simulink model "single_phase_WPT_v3"  (R2021a)
settings: Solver=FixedStepDiscrete  StartTime=0.0  StopTime=Tfinal  FixedStep=SampleTime  RelTol=1e-3
InitFcn:
  | param
values from neighbouring files (symbols this model uses):
  C_DCA = 1e-6    (= 1e-06)    [param.m]
  C_DCB = 1e-6    (= 1e-06)    [param.m]
  C_DCC = 1e-6    (= 1e-06)    [param.m]
  Cp = 28e-9    (= 2.8e-08)    [param.m]
  Cs = 120e-9    (= 1.2e-07)    [param.m]
  ESRA = 1e-7    (= 1e-07)    [param.m]
  ESRB = 1e-7    (= 1e-07)    [param.m]
  ESRC = 1e-7    (= 1e-07)    [param.m]
  f_motor = 50    [param.m]
  Lmotor = 30e-3    (= 0.03)    [param.m]
  Lp = 205e-6    (= 0.000205)    [param.m]
  Ls = 50e-6    (= 5e-05)    [param.m]
  LSource = 1e-9    (= 1e-09)    [param.m]
  M = 40e-6    (= 4e-05)    [param.m]
  ma = 0:0.01:1    [analitik_calculation.m]    (also in analytical_v2.m; param.m = 0.6)
  RL = 13    [param.m]
  Rmotor = 13    [param.m]
  RSource = 0.001    [param.m]
  SampleTime = 1e-8    (= 1e-08)    [param.m]
  Tfinal = 0.08    [param.m]
  VDC = 50    [param.m]
undefined symbols (not defined in the file or in its folder): ESLA, ESLB
libraries: spsSeriesRLCBranchLib x17, spsCurrentMeasurementLib x15, spsVoltageMeasurementLib x9, spsMosfetLib x6, spsTriangleGeneratorLib x3, spsDCVoltageSourceLib x1, eeStairGenerator x1, spsVariableResistorLib x1, spspowerguiLib x1
settings Model: Creator=enes_  LastModifiedBy=enes_
settings SolverCC: AlgebraicLoopSolver=TrustRegion
settings DataIOCC: ReturnWorkspaceOutputs=off
settings DebuggingCC: SFMachineParentedDataDiag=warning  ArithmeticOperatorsInVariantConditions=warning
settings SFSimCC: SimUseLocalCustomCode=off  CustomCodeUndefinedFunction=UseInterfaceOnly
settings RTWCC: RTWUseLocalCustomCode=off

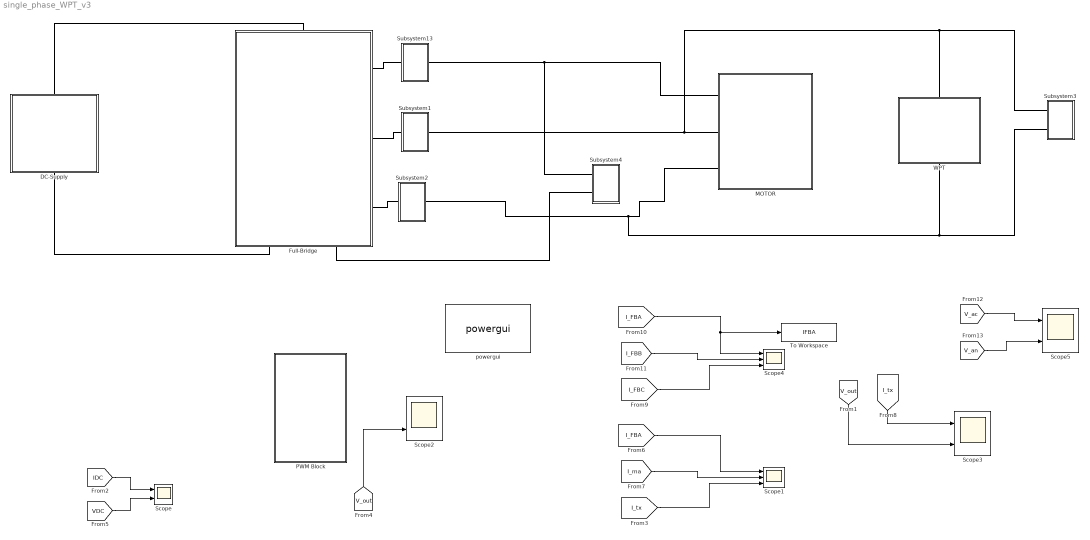
== system single_phase_WPT_v3 ==
  DC-Supply : Subsystem
  Full-Bridge : Subsystem
      settings: PortSchema="{\"entries\":[{\"content\":{\"sides\":[{\"content\":{\"connectorIds\":[]},\"type\":\"ConnectorPlacement.EquallySpacedRectSide\",\"uuid\":\"92c2640b-bb56-47f8-9c41-2323b38839f8\"},{\"content\":{\"connectorIds\":[\"RConn1\",\"RConn2\",\"RConn3\"],\"side\":\"RIGHT\"},\"type\":\"ConnectorPlacement.EquallySpacedRectSide\",\"uuid\":\"0b5c90a1-e2e1-4478-84c9-834496a6568e\"},{\"content\":{\"connectorIds\":[\"LConn1\"],\"side\":\"TOP\"},\"type\":\"ConnectorPlacement.EquallySpacedRectSide\",\"uuid\":\"1c803fb0-9096-4a7d-b495-aabd35d72306\"},{\"content\":{\"connectorIds\":[\"RConn4\",\"RConn5\"],\"side\":\"BOTTOM\"},\"type\":\"ConnectorPlacement.EquallySpacedRectSide\",\"uuid\":\"5a2d766c-8c3f-4943-ab0f-0e1988e2f8d8\"},{\"content\":{\"connectorIds\":[],\"side\":\"HIDDEN\"},\"type\":\"ConnectorPlacement.EquallySpacedRectSide\",\"uuid\":\"8868c32c-a67f-4887-a91d-dc24242eaee2\"}]},\"type\":\"ConnectorPlacement.EquallySpacedConnector\",\"uuid\":\"a3546067-6216-40b0-bae0-9d71271c5112\"}],\"packageUris\":[\"http://schema.mathworks.com/mf0/Connector/R2020b\"],\"version\":\"1.0\"}"
  MOTOR : Subsystem
      settings: PortSchema="{\"entries\":[{\"content\":{\"sides\":[{\"content\":{\"connectorIds\":[]},\"type\":\"ConnectorPlacement.EquallySpacedRectSide\",\"uuid\":\"27af0988-5d70-46f2-9f63-66e4679735d7\"},{\"content\":{\"connectorIds\":[],\"side\":\"RIGHT\"},\"type\":\"ConnectorPlacement.EquallySpacedRectSide\",\"uuid\":\"9d673fb6-38db-4110-ad66-771dcf318fba\"},{\"content\":{\"connectorIds\":[\"LConn1\",\"LConn2\",\"LConn3\"],\"side\":\"TOP\"},\"type\":\"ConnectorPlacement.EquallySpacedRectSide\",\"uuid\":\"44eb7bd4-c702-4f50-84c2-cb9d75020b5b\"},{\"content\":{\"connectorIds\":[],\"side\":\"HIDDEN\"},\"type\":\"ConnectorPlacement.EquallySpacedRectSide\",\"uuid\":\"ba714e9b-5efc-4dbb-add8-803f06cf9de0\"}]},\"type\":\"ConnectorPlacement.EquallySpacedConnector\",\"uuid\":\"a2219d53-abb4-437b-a840-c37860cec52f\"}],\"packageUris\":[\"http://schema.mathworks.com/mf0/Connector/R2020b\"],\"version\":\"1.0\"}"
  PWM Block : Subsystem
  Scope{,2..3,5} (4 alike) : Scope  NumInputPorts=2
  Scope1 : Scope  NumInputPorts=3
  Scope4 : Scope  NumInputPorts=3
  Subsystem1 : Subsystem
  Subsystem13 : Subsystem
  Subsystem2 : Subsystem
  Subsystem3 : Subsystem
  Subsystem4 : Subsystem
  To Workspace : ToWorkspace  VariableName=IFBA  SaveFormat=Timeseries  SampleTime=-1
  WPT : Subsystem
  powergui : spspowerguiLib/powergui  Priority=1  SimulationMode=Discrete  SampleTime=SampleTime  frequency=60  Iterations=50  frequencyindice=0  Pbase=100e6  ErrMax=1e-4  UnitsV=kV  UnitsW=MW  buscounter=0  FunctionMessages=off  echomessages=off  EnableUseOfTLC=off  CurrentSourceSwitches=off  DisableSnubberDevices=off  DisableRonSwitches=off  DisableVfSwitches=off  DisplayEquations=off  AutomaticDiscreteSolvers=off  SolverType=Tustin/Backward Euler (TBE)  Interpol=off  ExternalGateDelay=off  methode=off  Ts=100  x0status=blocks  SPID=on  SwTol=0  HookPort=off  NonlinearTolerance=1e-4  nMaxIteration=100  ContinueOnMaxIteration=off  RestoreLinks=warning  ResistiveCurrentMeasurement=off  Frange=[1e3:1e3:240e3]  Ylog=off  Xlog=on  ShowGrid=off  save=off  variable=ZData  structure=ScopeData2  ZoomFFT=off  StartTime=0.0005  cycles=800  DisplayStyle=1  fundamental=80000  FreqAxis=on  MaxFrequency=100e3  frequencyindicesteady=1  RmsSteady=1  display=off
  wires:
  [IDC] -> Scope/1
  [VDC] -> Scope/2
  [I_FBA] -> Scope1/1
  [I_ma] -> Scope1/2
  [I_tx] -> Scope1/3
  [V_out] -> Scope2/2
  ? -> Scope2/1
  [V_out] -> Scope3/2
  [I_tx] -> Scope3/1
  [I_FBB] -> Scope4/2
  [I_FBA] -> To Workspace/1, Scope4/1
  [I_FBC] -> Scope4/3
  [V_ac] -> Scope5/1
  [V_an] -> Scope5/2
  connections:
  DC-Supply/LConn1 -- Full-Bridge/LConn1
  DC-Supply/RConn1 -- Full-Bridge/RConn4
  Subsystem13/RConn1 -- Full-Bridge/RConn1
  MOTOR/LConn1 -- Subsystem13/LConn1 -- Subsystem4/LConn1
  Full-Bridge/RConn3 -- Subsystem2/RConn1
  Subsystem1/RConn1 -- Full-Bridge/RConn2
  WPT/LConn1 -- Subsystem3/LConn1 -- MOTOR/LConn2 -- Subsystem1/LConn1
  MOTOR/LConn3 -- WPT/RConn1 -- Subsystem3/LConn2 -- Subsystem2/LConn1
  Subsystem4/LConn2 -- Full-Bridge/RConn5

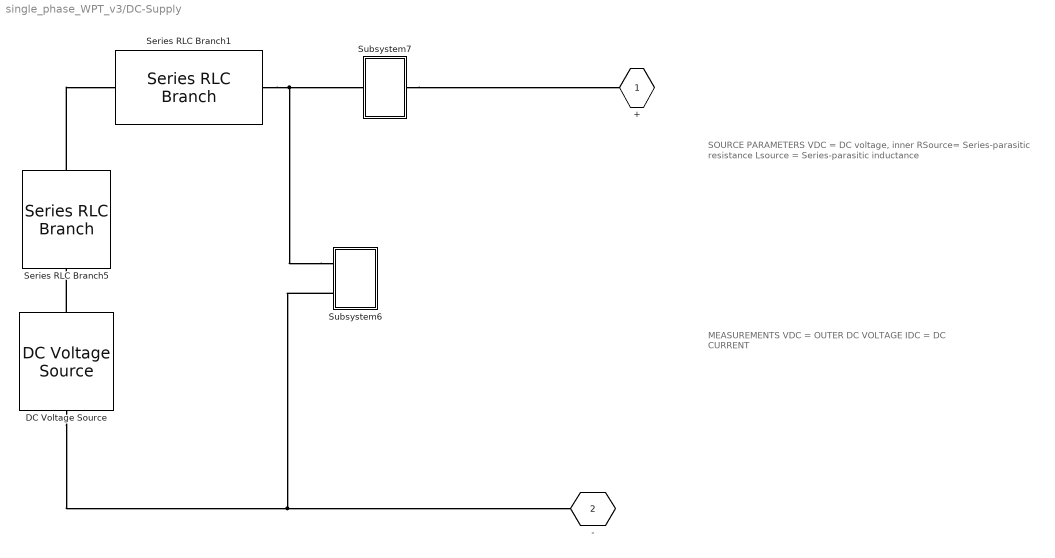
== system single_phase_WPT_v3/DC-Supply ==
  note: SOURCE PARAMETERS
      | VDC = DC voltage, inner
      | RSource= Series-parasitic resistance
      | Lsource = Series-parasitic inductance
  note: MEASUREMENTS
      | VDC = OUTER DC VOLTAGE
      | IDC = DC CURRENT
  DC Voltage Source : spsDCVoltageSourceLib/DC Voltage Source  Amplitude=VDC  Measurements=None
  Series RLC Branch1 : spsSeriesRLCBranchLib/Series RLC Branch  LConnTagsString=__new0  RConnTagsString=__new0  BranchType=L  Resistance=LSource  Inductance=LSource  SetiL0=off  InitialCurrent=0  Capacitance=0.01  Setx0=off  InitialVoltage=0  Measurements=None
  Series RLC Branch5 : spsSeriesRLCBranchLib/Series RLC Branch  LConnTagsString=__new0  RConnTagsString=__new0  BranchType=R  Resistance=RSource  Inductance=ESLA  SetiL0=off  InitialCurrent=0  Capacitance=0.01  Setx0=off  InitialVoltage=0  Measurements=None
  Subsystem6 : Subsystem
  Subsystem7 : Subsystem
  + : PMIOPort  Side=Left
  - : PMIOPort  Port=2  Side=Right
  connections:
  Series RLC Branch5/LConn1 -- Series RLC Branch1/RConn1
  DC Voltage Source/LConn1 -- Subsystem6/LConn2 -- -/RConn1
  Subsystem6/LConn1 -- Subsystem7/RConn1 -- Series RLC Branch1/LConn1
  DC Voltage Source/RConn1 -- Series RLC Branch5/RConn1
  Subsystem7/LConn1 -- +/RConn1

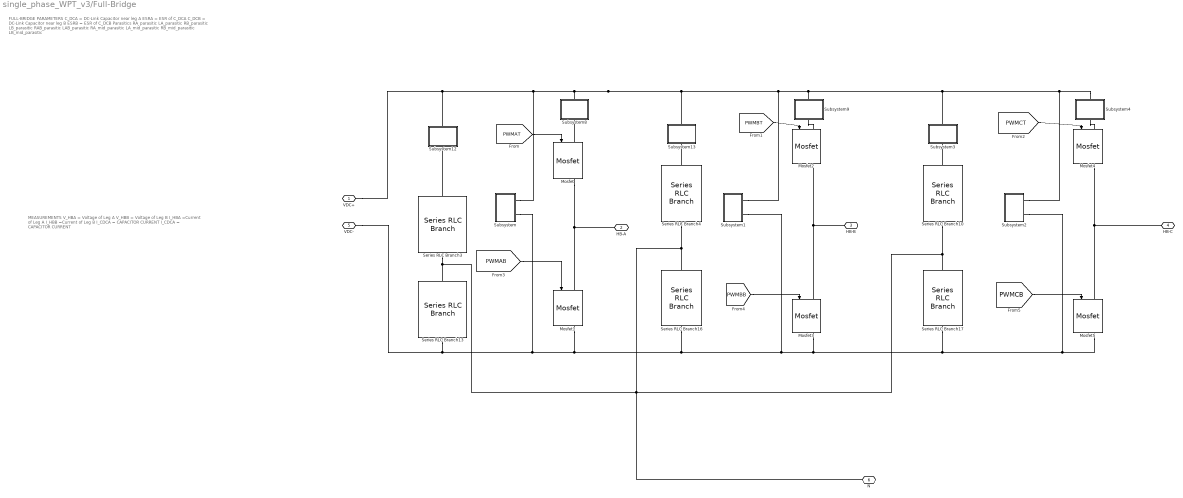
== system single_phase_WPT_v3/Full-Bridge ==
  note: MEASUREMENTS
      | V_HBA = Voltage of Leg A
      | V_HBB = Voltage of Leg B
      | I_HBA =Current of Leg A
      | I_HBB =Current of Leg B
      | I_CDCA = CAPACITOR CURRENT
      | I_CDCA = CAPACITOR CURRENT
  note: FULL-BRIDGE PARAMETERS
      | C_DCA = DC-Link Capacitor near leg A
      | ESRA = ESR of C_DCA
      | C_DCB = DC-Link Capacitor near leg B
      | ESRB = ESR of C_DCB
      | Parasitics
      | RA_parasitic
      | LA_parasitic
      | RB_parasitic
      | LB_parasitic
      | RAB_parasitic
      | LAB_parasitic
      | RA_mid_parasitic
      | LA_mid_parasitic
      | RB_mid_parasitic
      | LB_mid_parasitic
  Mosfet{,1..5} (6 alike) : spsMosfetLib/Mosfet  Ron=0.1  Lon=0  Rd=0.01  Vfd=0  IC=0  Rs=1e5  Cs=inf  Measurements=on
  Series RLC Branch10 : spsSeriesRLCBranchLib/Series RLC Branch  LConnTagsString=__new0  RConnTagsString=__new0  BranchType=C  Resistance=ESRC  Inductance=ESLB  SetiL0=off  InitialCurrent=0  Capacitance=C_DCC  Setx0=off  InitialVoltage=0  Measurements=None
  Series RLC Branch13 : spsSeriesRLCBranchLib/Series RLC Branch  LConnTagsString=__new0  RConnTagsString=__new0  BranchType=C  Resistance=ESRA  Inductance=ESLA  SetiL0=off  InitialCurrent=0  Capacitance=C_DCA  Setx0=off  InitialVoltage=0  Measurements=None
  Series RLC Branch16 : spsSeriesRLCBranchLib/Series RLC Branch  LConnTagsString=__new0  RConnTagsString=__new0  BranchType=C  Resistance=ESRB  Inductance=ESLB  SetiL0=off  InitialCurrent=0  Capacitance=C_DCB  Setx0=off  InitialVoltage=0  Measurements=None
  Series RLC Branch17 : spsSeriesRLCBranchLib/Series RLC Branch  LConnTagsString=__new0  RConnTagsString=__new0  BranchType=C  Resistance=ESRC  Inductance=ESLB  SetiL0=off  InitialCurrent=0  Capacitance=C_DCC  Setx0=off  InitialVoltage=0  Measurements=None
  Series RLC Branch3 : spsSeriesRLCBranchLib/Series RLC Branch  LConnTagsString=__new0  RConnTagsString=__new0  BranchType=C  Resistance=ESRA  Inductance=ESLA  SetiL0=off  InitialCurrent=0  Capacitance=C_DCA  Setx0=off  InitialVoltage=0  Measurements=None
  Series RLC Branch4 : spsSeriesRLCBranchLib/Series RLC Branch  LConnTagsString=__new0  RConnTagsString=__new0  BranchType=C  Resistance=ESRB  Inductance=ESLB  SetiL0=off  InitialCurrent=0  Capacitance=C_DCB  Setx0=off  InitialVoltage=0  Measurements=None
  Subsystem : Subsystem
  Subsystem1 : Subsystem
  Subsystem12 : Subsystem
  Subsystem13 : Subsystem
  Subsystem2 : Subsystem
  Subsystem3 : Subsystem
  Subsystem4 : Subsystem
  Subsystem8 : Subsystem
  Subsystem9 : Subsystem
  VDC+ : PMIOPort  Side=Left
  HB-A : PMIOPort  Port=2  Side=Right
  HB-B : PMIOPort  Port=3  Side=Right
  HB-C : PMIOPort  Port=4  Side=Right
  VDC- : PMIOPort  Port=5  Side=Right
  N : PMIOPort  Port=6  Side=Right
  wires:
  [PWMAB] -> Mosfet1/1
  [PWMAT] -> Mosfet/1
  [PWMBB] -> Mosfet3/1
  [PWMBT] -> Mosfet2/1
  [PWMCT] -> Mosfet4/1
  [PWMCB] -> Mosfet5/1
  connections:
  Subsystem4/RConn1 -- VDC+/RConn1 -- Subsystem12/RConn1 -- Subsystem/LConn1 -- Subsystem8/RConn1 -- Subsystem13/RConn1 -- Subsystem1/LConn1 -- Subsystem9/RConn1 -- Subsystem3/RConn1 -- Subsystem2/LConn1
  Subsystem9/LConn1 -- Mosfet2/LConn1
  Series RLC Branch4/LConn1 -- Subsystem13/LConn1
  Series RLC Branch3/LConn1 -- Subsystem12/LConn1
  HB-B/RConn1 -- Mosfet2/RConn1 -- Mosfet3/LConn1
  Mosfet/LConn1 -- Subsystem8/LConn1
  Subsystem2/LConn2 -- Mosfet5/RConn1 -- Series RLC Branch17/RConn1 -- Series RLC Branch16/RConn1 -- Series RLC Branch13/RConn1 -- VDC-/RConn1 -- Subsystem/LConn2 -- Mosfet1/RConn1 -- Subsystem1/LConn2 -- Mosfet3/RConn1
  HB-A/RConn1 -- Mosfet/RConn1 -- Mosfet1/LConn1
  Series RLC Branch10/LConn1 -- Subsystem3/LConn1
  HB-C/RConn1 -- Mosfet4/RConn1 -- Mosfet5/LConn1
  Subsystem4/LConn1 -- Mosfet4/LConn1
  Series RLC Branch10/RConn1 -- Series RLC Branch16/LConn1 -- Series RLC Branch4/RConn1 -- Series RLC Branch13/LConn1 -- Series RLC Branch3/RConn1 -- N/RConn1 -- Series RLC Branch17/LConn1

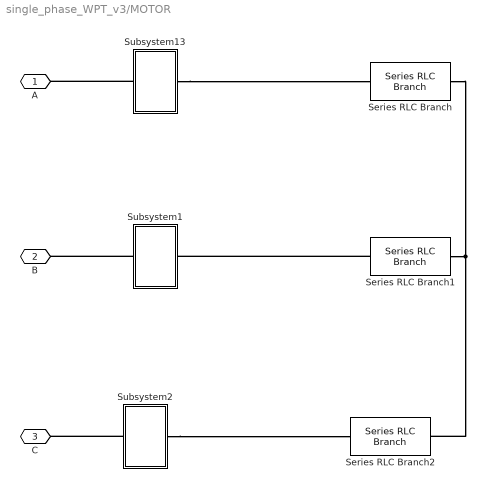
== system single_phase_WPT_v3/MOTOR ==
  Series RLC Branch : spsSeriesRLCBranchLib/Series RLC Branch  LConnTagsString=__new0  RConnTagsString=__new0  BranchType=RL  Resistance=Rmotor  Inductance=Lmotor  SetiL0=off  InitialCurrent=0  Capacitance=1e-6  Setx0=off  InitialVoltage=0  Measurements=None
  Series RLC Branch1 : spsSeriesRLCBranchLib/Series RLC Branch  LConnTagsString=__new0  RConnTagsString=__new0  BranchType=RL  Resistance=Rmotor  Inductance=Lmotor  SetiL0=off  InitialCurrent=0  Capacitance=1e-6  Setx0=off  InitialVoltage=0  Measurements=None
  Series RLC Branch2 : spsSeriesRLCBranchLib/Series RLC Branch  LConnTagsString=__new0  RConnTagsString=__new0  BranchType=RL  Resistance=Rmotor  Inductance=Lmotor  SetiL0=off  InitialCurrent=0  Capacitance=1e-6  Setx0=off  InitialVoltage=0  Measurements=None
  Subsystem1 : Subsystem
  Subsystem13 : Subsystem
  Subsystem2 : Subsystem
  A : PMIOPort  Side=Left
  B : PMIOPort  Port=2  Side=Left
  C : PMIOPort  Port=3  Side=Left
  connections:
  Subsystem13/LConn1 -- Series RLC Branch/LConn1
  Subsystem13/RConn1 -- A/RConn1
  Subsystem1/RConn1 -- B/RConn1
  Subsystem2/RConn1 -- C/RConn1
  Series RLC Branch1/LConn1 -- Subsystem1/LConn1
  Subsystem2/LConn1 -- Series RLC Branch2/LConn1
  Series RLC Branch/RConn1 -- Series RLC Branch2/RConn1 -- Series RLC Branch1/RConn1

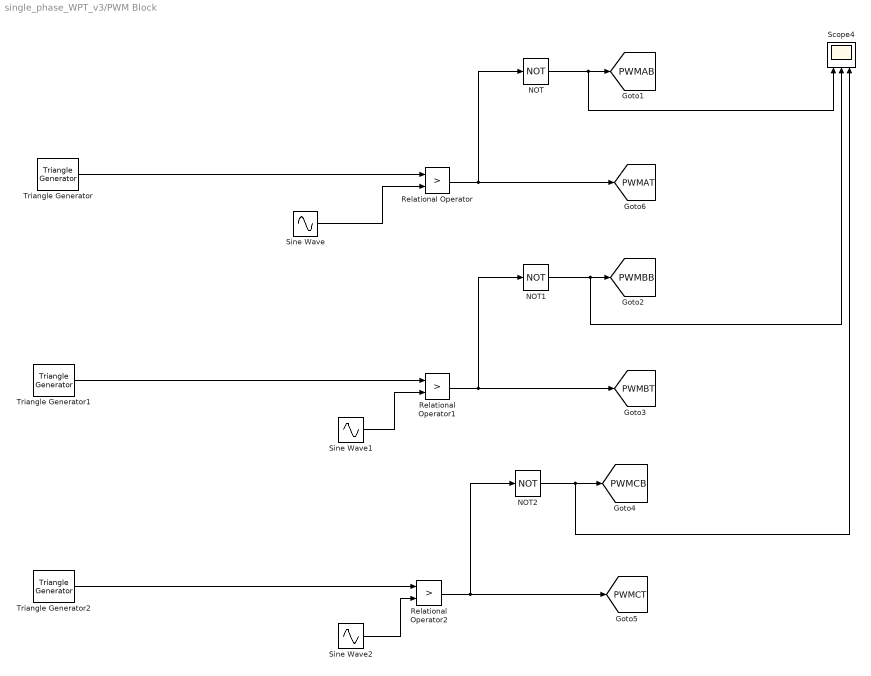
== system single_phase_WPT_v3/PWM Block ==
  NOT : Logic  Operator=NOT  IconShape=distinctive  AllPortsSameDT=off  OutDataTypeStr=boolean
  NOT1 : Logic  Operator=NOT  IconShape=distinctive  AllPortsSameDT=off  OutDataTypeStr=boolean
  NOT2 : Logic  Operator=NOT  IconShape=distinctive  AllPortsSameDT=off  OutDataTypeStr=boolean
  Relational Operator : RelationalOperator  Operator=>  OutDataTypeStr=boolean  RndMeth=Simplest
  Relational Operator1 : RelationalOperator  Operator=>  OutDataTypeStr=boolean  RndMeth=Simplest
  Relational Operator2 : RelationalOperator  Operator=>  OutDataTypeStr=boolean  RndMeth=Simplest
  Scope4 : Scope  NumInputPorts=3
  Sine Wave : Sin  Amplitude=ma  Frequency=f_motor*2*pi  SampleTime=0
  Sine Wave1 : Sin  Amplitude=ma  Frequency=f_motor*2*pi  Phase=-2*pi/3  SampleTime=0
  Sine Wave2 : Sin  Amplitude=ma  Frequency=f_motor*2*pi  Phase=2*pi/3  SampleTime=0
  Triangle Generator : spsTriangleGeneratorLib/Triangle Generator  Freq=80e3  Phase=0  Ts=SampleTime
  Triangle Generator1 : spsTriangleGeneratorLib/Triangle Generator  Freq=80e3  Phase=-120  Ts=SampleTime
  Triangle Generator2 : spsTriangleGeneratorLib/Triangle Generator  Freq=80e3  Phase=120  Ts=SampleTime
  tag scope: PWMAB=global, PWMAT=global, PWMBB=global, PWMBT=global, PWMCB=global, PWMCT=global
  wires:
  NOT/1 -> Scope4/1, [PWMAB]
  Relational Operator/1 -> NOT/1, [PWMAT]
  Relational Operator1/1 -> NOT1/1, [PWMBT]
  NOT2/1 -> [PWMCB], Scope4/3
  Relational Operator2/1 -> NOT2/1, [PWMCT]
  Sine Wave/1 -> Relational Operator/2
  Sine Wave2/1 -> Relational Operator2/2
  Sine Wave1/1 -> Relational Operator1/2
  NOT1/1 -> Scope4/2, [PWMBB]
  Triangle Generator/1 -> Relational Operator/1
  Triangle Generator1/1 -> Relational Operator1/1
  Triangle Generator2/1 -> Relational Operator2/1

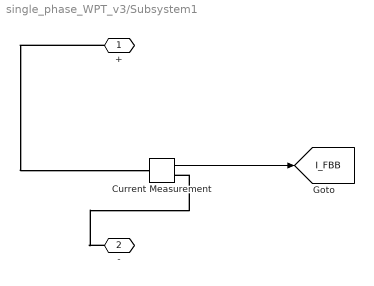
== system single_phase_WPT_v3/Subsystem1 ==
  Current Measurement : spsCurrentMeasurementLib/Current Measurement  PhasorSimulation=off  OutputType=Complex  PSBequivalent=0
  + : PMIOPort  Side=Right
  - : PMIOPort  Port=2  Side=Left
  tag scope: I_FBB=global
  wires:
  Current Measurement/1 -> [I_FBB]
  connections:
  +/RConn1 -- Current Measurement/LConn1
  -/RConn1 -- Current Measurement/RConn1

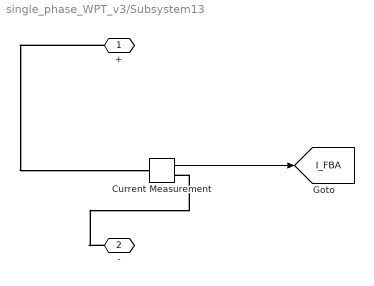
== system single_phase_WPT_v3/Subsystem13 ==
  Current Measurement : spsCurrentMeasurementLib/Current Measurement  PhasorSimulation=off  OutputType=Complex  PSBequivalent=0
  + : PMIOPort  Side=Right
  - : PMIOPort  Port=2  Side=Left
  tag scope: I_FBA=global
  wires:
  Current Measurement/1 -> [I_FBA]
  connections:
  +/RConn1 -- Current Measurement/LConn1
  -/RConn1 -- Current Measurement/RConn1

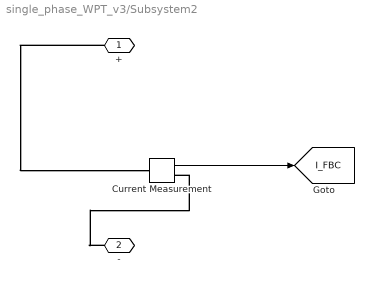
== system single_phase_WPT_v3/Subsystem2 ==
  Current Measurement : spsCurrentMeasurementLib/Current Measurement  PhasorSimulation=off  OutputType=Complex  PSBequivalent=0
  + : PMIOPort  Side=Right
  - : PMIOPort  Port=2  Side=Left
  tag scope: I_FBC=global
  wires:
  Current Measurement/1 -> [I_FBC]
  connections:
  +/RConn1 -- Current Measurement/LConn1
  -/RConn1 -- Current Measurement/RConn1

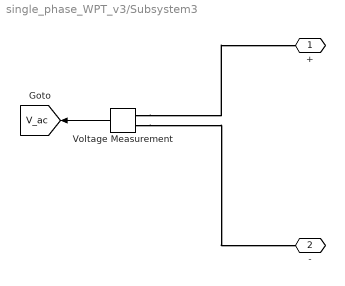
== system single_phase_WPT_v3/Subsystem3 ==
  Voltage Measurement : spsVoltageMeasurementLib/Voltage Measurement  PhasorSimulation=off  OutputType=Complex  PSBequivalent=0
  + : PMIOPort  Side=Left
  - : PMIOPort  Port=2  Side=Left
  tag scope: V_ac=global
  wires:
  Voltage Measurement/1 -> [V_ac]
  connections:
  Voltage Measurement/LConn1 -- +/RConn1
  Voltage Measurement/LConn2 -- -/RConn1

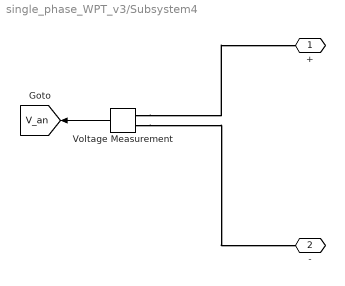
== system single_phase_WPT_v3/Subsystem4 ==
  Voltage Measurement : spsVoltageMeasurementLib/Voltage Measurement  PhasorSimulation=off  OutputType=Complex  PSBequivalent=0
  + : PMIOPort  Side=Left
  - : PMIOPort  Port=2  Side=Left
  tag scope: V_an=global
  wires:
  Voltage Measurement/1 -> [V_an]
  connections:
  Voltage Measurement/LConn1 -- +/RConn1
  Voltage Measurement/LConn2 -- -/RConn1

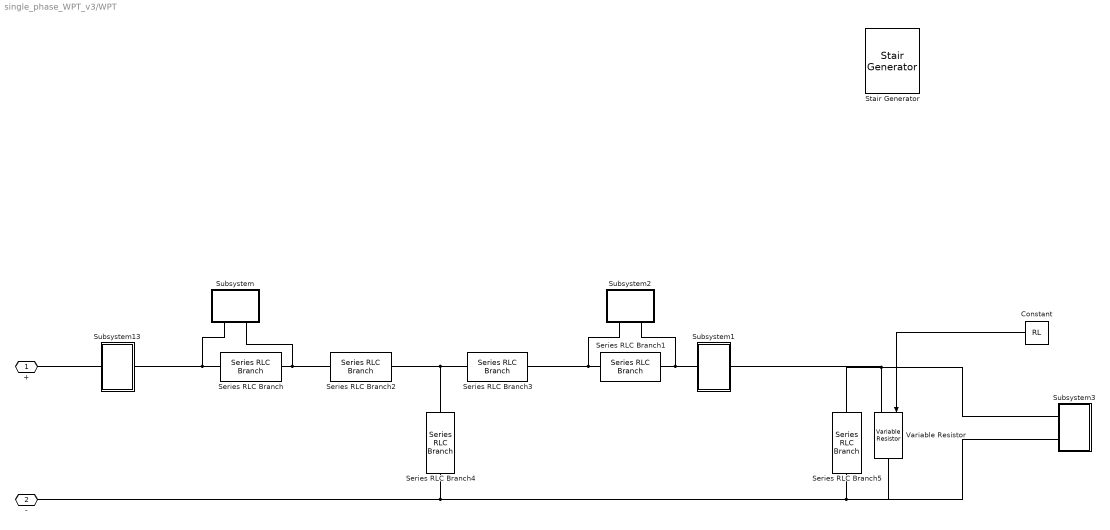
== system single_phase_WPT_v3/WPT ==
  Constant : Constant  Value=RL
  Series RLC Branch : spsSeriesRLCBranchLib/Series RLC Branch  LConnTagsString=__new0  RConnTagsString=__new0  BranchType=C  Resistance=1  Inductance=1e-3  SetiL0=off  InitialCurrent=0  Capacitance=Cp  Setx0=off  InitialVoltage=0  Measurements=None
  Series RLC Branch1 : spsSeriesRLCBranchLib/Series RLC Branch  LConnTagsString=__new0  RConnTagsString=__new0  BranchType=C  Resistance=1  Inductance=1e-3  SetiL0=off  InitialCurrent=0  Capacitance=Cs  Setx0=off  InitialVoltage=0  Measurements=None
  Series RLC Branch2 : spsSeriesRLCBranchLib/Series RLC Branch  LConnTagsString=__new0  RConnTagsString=__new0  BranchType=L  Resistance=1  Inductance=Lp-M  SetiL0=off  InitialCurrent=0  Capacitance=Cp  Setx0=off  InitialVoltage=0  Measurements=None
  Series RLC Branch3 : spsSeriesRLCBranchLib/Series RLC Branch  LConnTagsString=__new0  RConnTagsString=__new0  BranchType=L  Resistance=1  Inductance=Ls-M  SetiL0=off  InitialCurrent=0  Capacitance=Cp  Setx0=off  InitialVoltage=0  Measurements=None
  Series RLC Branch4 : spsSeriesRLCBranchLib/Series RLC Branch  LConnTagsString=__new0  RConnTagsString=__new0  BranchType=L  Resistance=1  Inductance=Lp-M  SetiL0=off  InitialCurrent=0  Capacitance=Cp  Setx0=off  InitialVoltage=0  Measurements=None
  Series RLC Branch5 : spsSeriesRLCBranchLib/Series RLC Branch  LConnTagsString=__new0  RConnTagsString=__new0  BranchType=R  Resistance=1e6  Inductance=Ls-M  SetiL0=off  InitialCurrent=0  Capacitance=Cp  Setx0=off  InitialVoltage=0  Measurements=None
  Stair Generator : eeStairGenerator/Stair Generator  LabelModeActiveChoice=Discrete  TimeInput=Tfinal*[0 1/4 2/4 3/4 ]  AmplitudeInput=RL*[1 1/2 0 100 ]  SampleTime=-1  RepeatPattern=off  OutDataTypeStr=double
      settings: SourceProductBaseCode=PS
  Subsystem : Subsystem
  Subsystem1 : Subsystem
  Subsystem13 : Subsystem
  Subsystem2 : Subsystem
  Subsystem3 : Subsystem
  Variable Resistor : spsVariableResistorLib/Variable Resistor  Rabsmin=1e-3
      settings: SourceProductBaseCode=PS
  + : PMIOPort  Side=Left
  - : PMIOPort  Port=2  Side=Right
  wires:
  Constant/1 -> Variable Resistor/1
  connections:
  Subsystem13/LConn1 -- Subsystem/LConn1 -- Series RLC Branch/LConn1
  Subsystem13/RConn1 -- +/RConn1
  Series RLC Branch2/LConn1 -- Subsystem/LConn2 -- Series RLC Branch/RConn1
  Series RLC Branch3/RConn1 -- Subsystem2/LConn1 -- Series RLC Branch1/RConn1
  Series RLC Branch4/LConn1 -- Series RLC Branch2/RConn1 -- Series RLC Branch3/LConn1
  Subsystem3/LConn1 -- Subsystem1/LConn1 -- Series RLC Branch5/LConn1 -- Variable Resistor/LConn1
  Subsystem1/RConn1 -- Subsystem2/LConn2 -- Series RLC Branch1/LConn1
  -/RConn1 -- Subsystem3/LConn2 -- Variable Resistor/RConn1 -- Series RLC Branch5/RConn1 -- Series RLC Branch4/RConn1

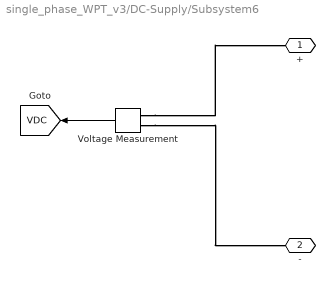
== system single_phase_WPT_v3/DC-Supply/Subsystem6 ==
  Voltage Measurement : spsVoltageMeasurementLib/Voltage Measurement  PhasorSimulation=off  OutputType=Complex  PSBequivalent=0
  + : PMIOPort  Side=Left
  - : PMIOPort  Port=2  Side=Left
  tag scope: VDC=global
  wires:
  Voltage Measurement/1 -> [VDC]
  connections:
  Voltage Measurement/LConn1 -- +/RConn1
  Voltage Measurement/LConn2 -- -/RConn1

== system single_phase_WPT_v3/DC-Supply/Subsystem7 ==
  Current Measurement : spsCurrentMeasurementLib/Current Measurement  PhasorSimulation=off  OutputType=Complex  PSBequivalent=0
  + : PMIOPort  Side=Right
  - : PMIOPort  Port=2  Side=Left
  tag scope: IDC=global
  wires:
  Current Measurement/1 -> [IDC]
  connections:
  +/RConn1 -- Current Measurement/LConn1
  -/RConn1 -- Current Measurement/RConn1

== system single_phase_WPT_v3/Full-Bridge/Subsystem ==
  Voltage Measurement : spsVoltageMeasurementLib/Voltage Measurement  PhasorSimulation=off  OutputType=Complex  PSBequivalent=0
  + : PMIOPort  Side=Left
  - : PMIOPort  Port=2  Side=Left
  tag scope: V_HBA=global
  wires:
  Voltage Measurement/1 -> [V_HBA]
  connections:
  Voltage Measurement/LConn1 -- +/RConn1
  Voltage Measurement/LConn2 -- -/RConn1

== system single_phase_WPT_v3/Full-Bridge/Subsystem1 ==
  Voltage Measurement : spsVoltageMeasurementLib/Voltage Measurement  PhasorSimulation=off  OutputType=Complex  PSBequivalent=0
  + : PMIOPort  Side=Left
  - : PMIOPort  Port=2  Side=Left
  tag scope: V_HBB=global
  wires:
  Voltage Measurement/1 -> [V_HBB]
  connections:
  Voltage Measurement/LConn1 -- +/RConn1
  Voltage Measurement/LConn2 -- -/RConn1

== system single_phase_WPT_v3/Full-Bridge/Subsystem12 ==
  Current Measurement : spsCurrentMeasurementLib/Current Measurement  PhasorSimulation=off  OutputType=Complex  PSBequivalent=0
  + : PMIOPort  Side=Right
  - : PMIOPort  Port=2  Side=Left
  tag scope: IC_DCA=global
  wires:
  Current Measurement/1 -> [IC_DCA]
  connections:
  +/RConn1 -- Current Measurement/LConn1
  -/RConn1 -- Current Measurement/RConn1

== system single_phase_WPT_v3/Full-Bridge/Subsystem13 ==
  Current Measurement : spsCurrentMeasurementLib/Current Measurement  PhasorSimulation=off  OutputType=Complex  PSBequivalent=0
  + : PMIOPort  Side=Right
  - : PMIOPort  Port=2  Side=Left
  tag scope: I_CDCB=global
  wires:
  Current Measurement/1 -> [I_CDCB]
  connections:
  +/RConn1 -- Current Measurement/LConn1
  -/RConn1 -- Current Measurement/RConn1

== system single_phase_WPT_v3/Full-Bridge/Subsystem2 ==
  Voltage Measurement : spsVoltageMeasurementLib/Voltage Measurement  PhasorSimulation=off  OutputType=Complex  PSBequivalent=0
  + : PMIOPort  Side=Left
  - : PMIOPort  Port=2  Side=Left
  tag scope: V_HBC=global
  wires:
  Voltage Measurement/1 -> [V_HBC]
  connections:
  Voltage Measurement/LConn1 -- +/RConn1
  Voltage Measurement/LConn2 -- -/RConn1

== system single_phase_WPT_v3/Full-Bridge/Subsystem3 ==
  Current Measurement : spsCurrentMeasurementLib/Current Measurement  PhasorSimulation=off  OutputType=Complex  PSBequivalent=0
  + : PMIOPort  Side=Right
  - : PMIOPort  Port=2  Side=Left
  tag scope: I_CDCC=global
  wires:
  Current Measurement/1 -> [I_CDCC]
  connections:
  +/RConn1 -- Current Measurement/LConn1
  -/RConn1 -- Current Measurement/RConn1

== system single_phase_WPT_v3/Full-Bridge/Subsystem4 ==
  Current Measurement : spsCurrentMeasurementLib/Current Measurement  PhasorSimulation=off  OutputType=Complex  PSBequivalent=0
  + : PMIOPort  Side=Right
  - : PMIOPort  Port=2  Side=Left
  tag scope: I_HBC=global
  wires:
  Current Measurement/1 -> [I_HBC]
  connections:
  +/RConn1 -- Current Measurement/LConn1
  -/RConn1 -- Current Measurement/RConn1

== system single_phase_WPT_v3/Full-Bridge/Subsystem8 ==
  Current Measurement : spsCurrentMeasurementLib/Current Measurement  PhasorSimulation=off  OutputType=Complex  PSBequivalent=0
  + : PMIOPort  Side=Right
  - : PMIOPort  Port=2  Side=Left
  tag scope: I_HBA=global
  wires:
  Current Measurement/1 -> [I_HBA]
  connections:
  +/RConn1 -- Current Measurement/LConn1
  -/RConn1 -- Current Measurement/RConn1

== system single_phase_WPT_v3/Full-Bridge/Subsystem9 ==
  Current Measurement : spsCurrentMeasurementLib/Current Measurement  PhasorSimulation=off  OutputType=Complex  PSBequivalent=0
  + : PMIOPort  Side=Right
  - : PMIOPort  Port=2  Side=Left
  tag scope: I_HBB=global
  wires:
  Current Measurement/1 -> [I_HBB]
  connections:
  +/RConn1 -- Current Measurement/LConn1
  -/RConn1 -- Current Measurement/RConn1

== system single_phase_WPT_v3/MOTOR/Subsystem1 ==
  Current Measurement : spsCurrentMeasurementLib/Current Measurement  PhasorSimulation=off  OutputType=Complex  PSBequivalent=0
  + : PMIOPort  Side=Right
  - : PMIOPort  Port=2  Side=Left
  tag scope: I_mb=global
  wires:
  Current Measurement/1 -> [I_mb]
  connections:
  +/RConn1 -- Current Measurement/LConn1
  -/RConn1 -- Current Measurement/RConn1

== system single_phase_WPT_v3/MOTOR/Subsystem13 ==
  Current Measurement : spsCurrentMeasurementLib/Current Measurement  PhasorSimulation=off  OutputType=Complex  PSBequivalent=0
  + : PMIOPort  Side=Right
  - : PMIOPort  Port=2  Side=Left
  tag scope: I_ma=global
  wires:
  Current Measurement/1 -> [I_ma]
  connections:
  +/RConn1 -- Current Measurement/LConn1
  -/RConn1 -- Current Measurement/RConn1

== system single_phase_WPT_v3/MOTOR/Subsystem2 ==
  Current Measurement : spsCurrentMeasurementLib/Current Measurement  PhasorSimulation=off  OutputType=Complex  PSBequivalent=0
  + : PMIOPort  Side=Right
  - : PMIOPort  Port=2  Side=Left
  tag scope: I_mc=global
  wires:
  Current Measurement/1 -> [I_mc]
  connections:
  +/RConn1 -- Current Measurement/LConn1
  -/RConn1 -- Current Measurement/RConn1

== system single_phase_WPT_v3/WPT/Subsystem ==
  Voltage Measurement : spsVoltageMeasurementLib/Voltage Measurement  PhasorSimulation=off  OutputType=Complex  PSBequivalent=0
  + : PMIOPort  Side=Left
  - : PMIOPort  Port=2  Side=Left
  tag scope: V_txCap=global
  wires:
  Voltage Measurement/1 -> [V_txCap]
  connections:
  Voltage Measurement/LConn1 -- +/RConn1
  Voltage Measurement/LConn2 -- -/RConn1

== system single_phase_WPT_v3/WPT/Subsystem1 ==
  Current Measurement : spsCurrentMeasurementLib/Current Measurement  PhasorSimulation=off  OutputType=Complex  PSBequivalent=0
  + : PMIOPort  Side=Right
  - : PMIOPort  Port=2  Side=Left
  tag scope: I_rx=global
  wires:
  Current Measurement/1 -> [I_rx]
  connections:
  +/RConn1 -- Current Measurement/LConn1
  -/RConn1 -- Current Measurement/RConn1

== system single_phase_WPT_v3/WPT/Subsystem13 ==
  Current Measurement : spsCurrentMeasurementLib/Current Measurement  PhasorSimulation=off  OutputType=Complex  PSBequivalent=0
  + : PMIOPort  Side=Right
  - : PMIOPort  Port=2  Side=Left
  tag scope: I_tx=global
  wires:
  Current Measurement/1 -> [I_tx]
  connections:
  +/RConn1 -- Current Measurement/LConn1
  -/RConn1 -- Current Measurement/RConn1

== system single_phase_WPT_v3/WPT/Subsystem2 ==
  Voltage Measurement : spsVoltageMeasurementLib/Voltage Measurement  PhasorSimulation=off  OutputType=Complex  PSBequivalent=0
  + : PMIOPort  Side=Left
  - : PMIOPort  Port=2  Side=Left
  tag scope: V_rxCap=global
  wires:
  Voltage Measurement/1 -> [V_rxCap]
  connections:
  Voltage Measurement/LConn1 -- +/RConn1
  Voltage Measurement/LConn2 -- -/RConn1

== system single_phase_WPT_v3/WPT/Subsystem3 ==
  Voltage Measurement : spsVoltageMeasurementLib/Voltage Measurement  PhasorSimulation=off  OutputType=Complex  PSBequivalent=0
  + : PMIOPort  Side=Left
  - : PMIOPort  Port=2  Side=Left
  tag scope: V_out=global
  wires:
  Voltage Measurement/1 -> [V_out]
  connections:
  Voltage Measurement/LConn1 -- +/RConn1
  Voltage Measurement/LConn2 -- -/RConn1
